simulink model "simulink_ex8"  (R2020a)
settings: Solver=FixedStepAuto  StartTime=0.0  StopTime=500  FixedStep=1e-3  RelTol=1e-3
libraries: simulink x1
settings Model: Creator=debora  LastModifiedBy=debora

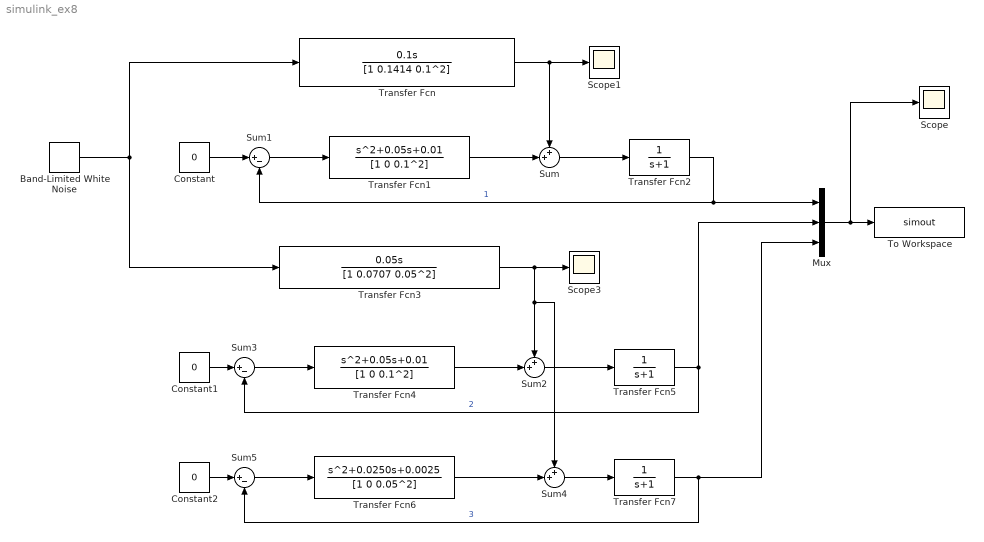
== system simulink_ex8 ==
  Band-Limited White Noise : simulink/Sources/Band-Limited White Noise  Cov=25  Ts=0.1  seed=[23341]
  Constant : Constant  Value=0
  Constant1 : Constant  Value=0
  Constant2 : Constant  Value=0
  Mux : Mux  Inputs=3
  Scope : Scope
  Scope1 : Scope
  Scope3 : Scope
  Sum : Sum  Inputs=++|
  Sum1 : Sum  Inputs=|+-
  Sum2 : Sum  Inputs=++|
  Sum3 : Sum  Inputs=|+-
  Sum4 : Sum  Inputs=++|
  Sum5 : Sum  Inputs=|+-
  To Workspace : ToWorkspace  VariableName=simout  SaveFormat=Timeseries  SampleTime=-1
  Transfer Fcn : TransferFcn  Numerator=[0.1 0]  Denominator=[1 0.1414 0.1^2]
  Transfer Fcn1 : TransferFcn  Numerator=[1 0.05 0.01]  Denominator=[1 0 0.1^2]
  Transfer Fcn2 : TransferFcn  Denominator=[1 1]
  Transfer Fcn3 : TransferFcn  Numerator=[0.05 0]  Denominator=[1 0.0707 0.05^2]
  Transfer Fcn4 : TransferFcn  Numerator=[1 0.05 0.01]  Denominator=[1 0 0.1^2]
  Transfer Fcn5 : TransferFcn  Denominator=[1 1]
  Transfer Fcn6 : TransferFcn  Numerator="[1 0.0250    0.0025]"  Denominator=[1 0 0.05^2]
  Transfer Fcn7 : TransferFcn  Denominator=[1 1]
  wires:
  Transfer Fcn/1 -> Sum/1, Scope1/1
  Transfer Fcn1/1 -> Sum/2
  Sum/1 -> Transfer Fcn2/1
  Transfer Fcn2/1 -> Mux/1, Sum1/2  "1"
  Constant/1 -> Sum1/1
  Sum1/1 -> Transfer Fcn1/1
  Transfer Fcn3/1 -> Scope3/1, Sum4/1, Sum2/1
  Band-Limited White Noise/1 -> Transfer Fcn3/1, Transfer Fcn/1
  Sum2/1 -> Transfer Fcn5/1
  Transfer Fcn4/1 -> Sum2/2
  Transfer Fcn5/1 -> Mux/2, Sum3/2  "2"
  Sum3/1 -> Transfer Fcn4/1
  Constant1/1 -> Sum3/1
  Constant2/1 -> Sum5/1
  Sum5/1 -> Transfer Fcn6/1
  Transfer Fcn6/1 -> Sum4/2
  Sum4/1 -> Transfer Fcn7/1
  Transfer Fcn7/1 -> Mux/3, Sum5/2  "3"
  Mux/1 -> Scope/1, To Workspace/1
